simulink model "t_oscillateur"  (R2015a)
settings: Solver=ode45  StartTime=0.0  StopTime=0.1  MaxStep=1e-6  MinStep=1e-10  RelTol=1e-3
values from neighbouring files (symbols this model uses):
  denC = [R*C 1]    [fp_oscillateur.m]    (also in tp_oscillateur.m)
  denG = [1/(2*pi*f0) 1]    [fp_oscillateur.m]    (also in tp_oscillateur.m)
  K = 1e-6    (= 1e-06)    [BodeTest.m]    (also in fp_oscillateur.m = 0.0001; test_multiple.m = linspace(0,1e-4,50); tp_oscillateur.m = 0.0001)
  numC = 1    [fp_oscillateur.m]    (also in tp_oscillateur.m)
  numG = A0    (= 100000)    [fp_oscillateur.m]    (also in tp_oscillateur.m)
settings Model: Creator=mserrari  LastModifiedBy=mserrari
settings SolverCC: InitialStep=1e-8

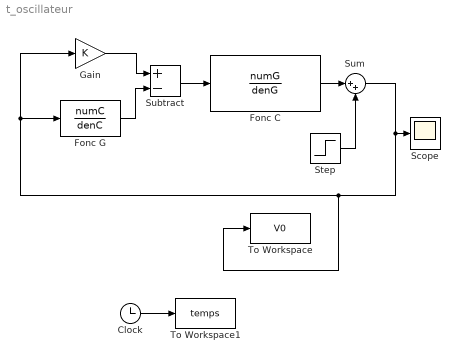
== system t_oscillateur ==
  Clock : Clock
  Fonc C : TransferFcn  Numerator=numG  Denominator=denG
  Fonc G : TransferFcn  Numerator=numC  Denominator=denC
  Gain : Gain  Gain=K
  Scope : Scope
  Step : Step  Time=0.05  After=0.01  SampleTime=0
  Subtract : Sum  Inputs=+-
  Sum : Sum  Inputs=|++
  To Workspace : ToWorkspace  VariableName=V0  SampleTime=-1
  To Workspace1 : ToWorkspace  VariableName=temps  SampleTime=-1
  wires:
  Fonc G/1 -> Subtract/2
  Gain/1 -> Subtract/1
  Subtract/1 -> Fonc C/1
  Step/1 -> Sum/2
  Fonc C/1 -> Sum/1
  Sum/1 -> To Workspace/1, Gain/1, Fonc G/1, Scope/1
  Clock/1 -> To Workspace1/1
